simulink model "controllingRC"  (R2016a)
settings: Solver=FixedStepAuto  StartTime=0.0  StopTime=inf  RelTol=1e-3
libraries: arduinolib x7
settings Model: SimulationMode=external  ExtModeTrigDuration=2  Creator=pc  LastModifiedBy=pc
settings OptimizationCC: OptimizeModelRefInitCode=on  LifeSpan=Inf  MaxStackSize=64
settings HardwareCC: ProdBitPerInt=16  ProdBitPerPointer=16  ProdLargestAtomicFloat=None  ProdWordSize=8  ProdHWDeviceType=Atmel->AVR
settings RTWCC: SystemTargetFile=ert.tlc  HardwareBoard=Arduino Uno  TemplateMakefile=ert_default_tmf  GenerateReport=on  Toolchain=Arduino AVR v1.6.1  BuildConfiguration=Faster Runs  IncludeHyperlinkInReport=on  LaunchReport=on  GenerateTraceInfo=on  GenerateTraceReport=on  GenerateTraceReportSl=on  GenerateTraceReportSf=on  GenerateTraceReportEml=on
settings CodeAppCC: ForceParamTrailComments=on  IgnoreCustomStorageClasses=off  OperatorAnnotations=on  SimulinkDataObjDesc=on  SFDataObjDesc=on  MATLABFcnDesc=on  InsertBlockDesc=on  MATLABSourceComments=on
settings ERTTargetCC: SupportContinuousTime=on  SupportVariableSizeSignals=on

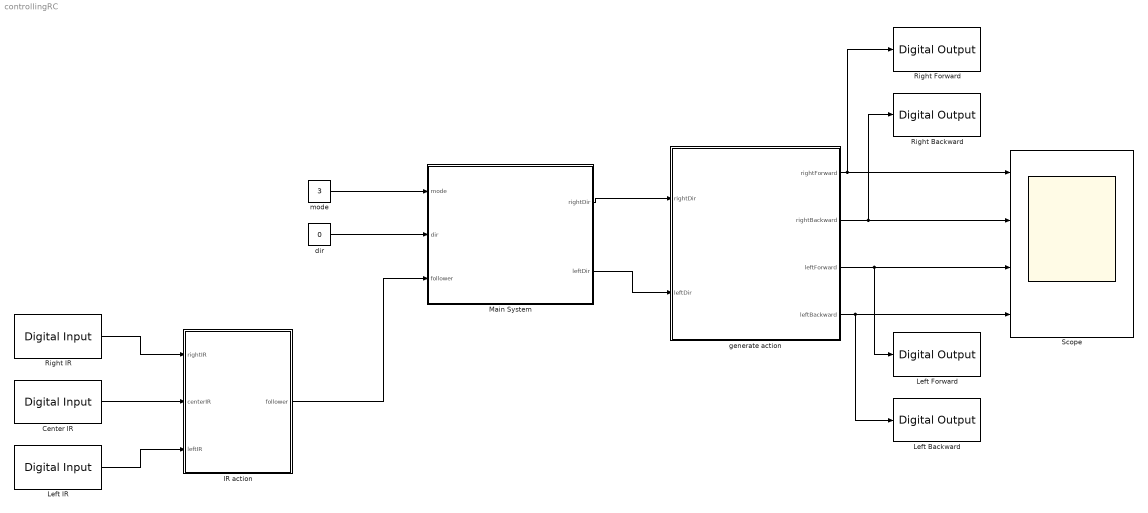
== system controllingRC ==
  Center IR : arduinolib/Digital Input  pinNumber=5  sampleTime=1  blockPlatform=arduino
  IR action : MATLAB Function  TreatAsAtomicUnit=on
  Left Backward : arduinolib/Digital Output  pinNumber=9  blockPlatform=arduino
  Left Forward : arduinolib/Digital Output  pinNumber=8  blockPlatform=arduino
  Left IR : arduinolib/Digital Input  pinNumber=4  sampleTime=1  blockPlatform=arduino
  Main System : Stateflow chart  TreatAsAtomicUnit=on
  Right Backward : arduinolib/Digital Output  pinNumber=11  blockPlatform=arduino
  Right Forward : arduinolib/Digital Output  pinNumber=10  blockPlatform=arduino
  Right IR : arduinolib/Digital Input  pinNumber=3  sampleTime=1  blockPlatform=arduino
  Scope : Scope  NumInputPorts=4
  dir : Constant  Value=0
  generate action : MATLAB Function  TreatAsAtomicUnit=on
  mode : Constant  Value=3
  wires:
  mode/1 -> Main System/1(mode)
  dir/1 -> Main System/2(dir)
  Main System/1(rightDir) -> generate action/1(rightDir)
  Main System/2(leftDir) -> generate action/2(leftDir)
  generate action/4(leftBackward) -> Left Backward/1, Scope/4
  generate action/3(leftForward) -> Left Forward/1, Scope/3
  generate action/2(rightBackward) -> Right Backward/1, Scope/2
  generate action/1(rightForward) -> Right Forward/1, Scope/1
  Right IR/1 -> IR action/1(rightIR)
  Center IR/1 -> IR action/2(centerIR)
  Left IR/1 -> IR action/3(leftIR)
  IR action/1(follower) -> Main System/3(follower)

== stateflow chart controllingRC/Main System ==
  state rightIR
    entry: rightDir = 0
    leftDir = 1
  state lineFollower
    entry: rightDir = 0
    leftDir = 0
  state centerIR
    entry: rightDir = 1
    leftDir = 1
  state leftIR
    entry: rightDir = 1
    leftDir = 0
  state mainMenu
    entry: rightDir = 0
    leftDir = 0
  state forward
    entry: rightDir = 1
    leftDir =1
  state right
    entry: rightDir = 0
    leftDir =1
  state left
    entry: rightDir = 1
    leftDir = 0
  state exitMode
    entry: rightDir = 0
    leftDir = 0
  state backward
    entry: rightDir = -1
    leftDir = -1
  state manualControl
    entry: rightDir = 0
    leftDir = 0
  lineFollower -> rightIR [order 2] : [follower == 2 && dir == 1]
  rightIR -> lineFollower : [follower ~= 2 || mode == 0 || dir == 0]
  lineFollower -> centerIR [order 3] : [follower == 1 && dir == 1]
  mainMenu -> lineFollower [order 1] : [mode ==1 ]
  centerIR -> lineFollower : [follower ~= 1 || mode == 0 || dir == 0]
  lineFollower -> mainMenu [order 1] : [mode ~= 1]
  lineFollower -> leftIR [order 4] : [follower == 3 && dir == 1]
  leftIR -> lineFollower : [follower ~= 3 || mode == 0 || dir == 0]
  (default) -> mainMenu [order 1]
  manualControl -> mainMenu [order 2] : [mode ~= 2]
  forward -> right [order 2] : [dir == 3]
  forward -> manualControl [order 1] : [ mode == 0 || dir == 0]
  mainMenu -> exitMode [order 3] : [mode == 3]
  mainMenu -> manualControl [order 2] : [mode == 2]
  manualControl -> forward [order 5] : [dir == 1]
  right -> forward [order 2] : [dir == 1]
  forward -> left [order 4] : [dir == 4]
  left -> forward [order 2] : [dir == 1]
  backward -> forward [order 3] : [dir == 1]
  forward -> backward [order 3] : [dir == 2]
  manualControl -> left [order 3] : [dir == 4]
  right -> manualControl [order 1] : [ mode == 0 || dir == 0]
  right -> left [order 4] : [dir == 4]
  left -> right [order 3] : [dir == 3]
  manualControl -> right [order 1] : [dir == 3]
  right -> backward [order 3] : [dir == 2]
  backward -> right [order 2] : [dir == 3]
  left -> manualControl [order 1] : [mode == 0 || dir == 0]
  backward -> left [order 4] : [dir == 4]
  left -> backward [order 4] : [dir == 2]
  backward -> manualControl [order 1] : [ mode == 0 || dir == 0]
  manualControl -> backward [order 4] : [dir == 2]
  (default) -> manualControl [order 2]
  data: mode input; dir input; rightDir output; leftDir output; follower input

== matlab function controllingRC/generate action ==
  data: rightForward output; rightBackward output; rightDir input; leftDir input; leftForward output; leftBackward output
function [rightForward,rightBackward,leftForward,leftBackward] = generateAction(rightDir,leftDir)
%#codegen

    if (rightDir == 1 && leftDir == 1 )
        rightForward = 5;
        rightBackward = 0;
        leftForward = 5;
        leftBackward = 0;
    elseif (rightDir == 1 && leftDir == 0)
        rightForward = 5;
        rightBackward = 0;
        leftForward = 0;
        leftBackward = 0;
    elseif (rightDir == 0 && leftDir == 1)
        rightForward = 0;
        rightBackward = 0;
        leftForward = 5;
        leftBackward = 0;

    elseif (rightDir == -1 && leftDir == -1)
        rightForward = 0;
        rightBackward = 5;
        leftForward = 0;
        leftBackward = 5;
    else
        rightForward = 0;
        rightBackward = 0;
        leftForward = 0;
        leftBackward = 0;
    end
        

end

== matlab function controllingRC/IR action ==
  data: rightIR input; follower output; centerIR input; leftIR input
function follower = determineFollowing(rightIR,centerIR,leftIR)
%#codegen
% 1 for black, 0 for white
    if (rightIR == 1 && centerIR == 0 && leftIR == 0 )
        follower = 2;
    elseif (rightIR == 0 && centerIR == 0 && leftIR == 1)
        follower = 3;
    else
        follower = 1;
    end

end
